simulink model "Feedforward_variations_Feb25_2017"  (R2016a)
settings: Solver=ode4  StartTime=0.0  StopTime=5  FixedStep=0.0001  RelTol=1e-3
values from neighbouring files (symbols this model uses):
  k = 10    [ff_demo_set_up.m]
  Kf = 1/(p+k)    (= 0.0666666666667)    [ff_demo_set_up.m]
  p = 5    [ff_demo_set_up.m]
libraries: simulink x4
settings Model: Creator=tac29  LastModifiedBy=DR_C

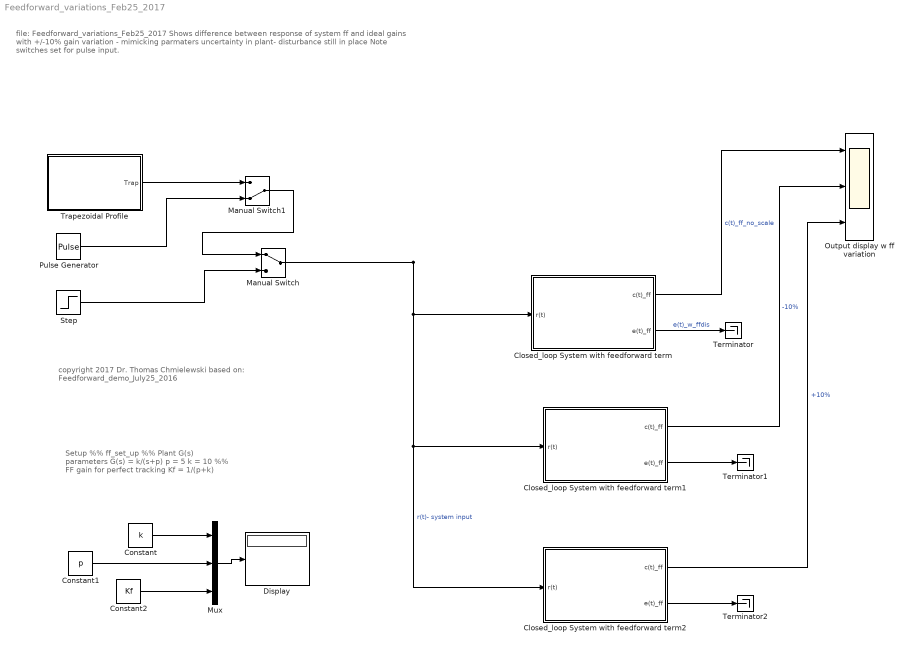
== system Feedforward_variations_Feb25_2017 ==
  note: file: Feedforward_variations_Feb25_2017
      | Shows difference between response of system ff and ideal gains with +/-10% gain variation - mimicking parmaters uncertainty in plant- disturbance still in place
      | Note switches set for pulse input.
  note: Setup
      | %% ff_set_up
      | %% Plant G(s) parameters   G(s) = k/(s+p)
      | p = 5
      | k = 10
      |
      | %% FF gain for perfect tracking
      | Kf = 1/(p+k)
  note: copyright 2017
      | Dr. Thomas Chmielewski
      | based on:
      | Feedforward_demo_July25_2016
  Closed_loop System with feedforward term : Subsystem
  Closed_loop System with feedforward term1 : Subsystem
  Closed_loop System with feedforward term2 : Subsystem
  Constant : Constant  Value=k
  Constant1 : Constant  Value=p
  Constant2 : Constant  Value=Kf
  Display : Display
  Manual Switch : ManualSwitch
  Manual Switch1 : ManualSwitch  CurrentSetting=0
  Mux : Mux  Inputs=3
  Output display w ff variation : Scope  NumInputPorts=3
  Pulse Generator : DiscretePulseGenerator  PulseType=Time based  Period=1  PulseWidth=50
  Step : Step  Time=0  SampleTime=0
  Terminator : Terminator
  Terminator1 : Terminator
  Terminator2 : Terminator
  Trapezoidal Profile : Subsystem
  wires:
  Step/1 -> Manual Switch/2
  Manual Switch/1 -> Closed_loop System with feedforward term2/1(r(t)), Closed_loop System with feedforward term1/1(r(t)), Closed_loop System with feedforward term/1(r(t))  "r(t)- system input"
  Mux/1 -> Display/1
  Constant2/1 -> Mux/3
  Constant1/1 -> Mux/2
  Constant/1 -> Mux/1
  Manual Switch1/1 -> Manual Switch/1
  Pulse Generator/1 -> Manual Switch1/2
  Trapezoidal Profile/1(Trap) -> Manual Switch1/1
  Closed_loop System with feedforward term/1(c(t)_ff) -> Output display w ff variation/1  "c(t)_ff_no_scale"
  Closed_loop System with feedforward term1/1(c(t)_ff) -> Output display w ff variation/2  "-10%"
  Closed_loop System with feedforward term2/1(c(t)_ff) -> Output display w ff variation/3  "+10%"
  Closed_loop System with feedforward term2/2(e(t)_ff) -> Terminator2/1
  Closed_loop System with feedforward term1/2(e(t)_ff) -> Terminator1/1
  Closed_loop System with feedforward term/2(e(t)_ff) -> Terminator/1  "e(t)_w_ffdis"

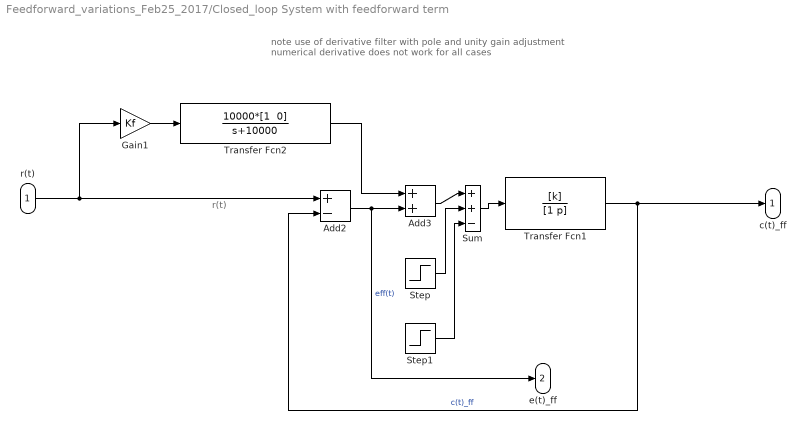
== system Feedforward_variations_Feb25_2017/Closed_loop System with feedforward term ==
  note: note use of derivative filter with pole and unity gain adjustment
      | numerical derivative does not work for all cases
  note: r(t)
  r(t) : Inport
  Add2 : Sum  Inputs=+-
  Add3 : Sum
  Gain1 : Gain  Gain=Kf
  Step : Step  Time=0  SampleTime=0
  Step1 : Step  Time=0  SampleTime=0
  Sum : Sum  Inputs=|++-
  Transfer Fcn1 : TransferFcn  Numerator=[k]  Denominator=[1 p]
  Transfer Fcn2 : TransferFcn  Numerator="10000*[1  0]"  Denominator=[1 10000]
  c(t)_ff : Outport
  e(t)_ff : Outport  Port=2
  wires:
  Add2/1 -> e(t)_ff/1, Add3/2  "eff(t)"
  Gain1/1 -> Transfer Fcn2/1
  Transfer Fcn1/1 -> c(t)_ff/1, Add2/2  "c(t)_ff"
  Transfer Fcn2/1 -> Add3/1
  r(t)/1 -> Add2/1, Gain1/1
  Add3/1 -> Sum/1
  Sum/1 -> Transfer Fcn1/1
  Step/1 -> Sum/2
  Step1/1 -> Sum/3

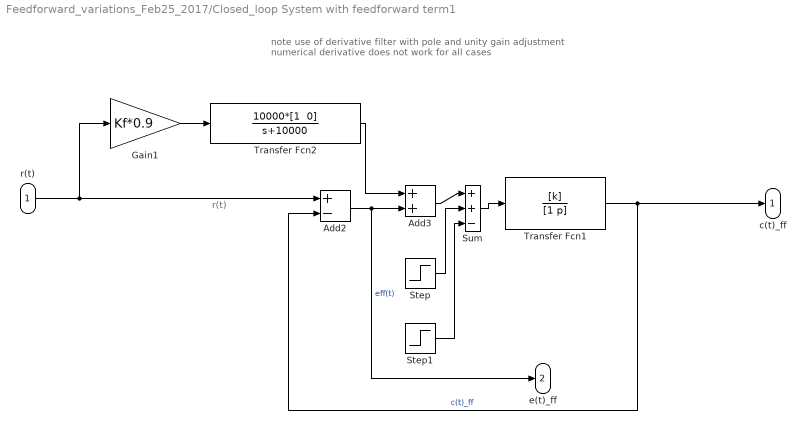
== system Feedforward_variations_Feb25_2017/Closed_loop System with feedforward term1 ==
  note: note use of derivative filter with pole and unity gain adjustment
      | numerical derivative does not work for all cases
  note: r(t)
  r(t) : Inport
  Add2 : Sum  Inputs=+-
  Add3 : Sum
  Gain1 : Gain  Gain=Kf*0.9
  Step : Step  Time=0  SampleTime=0
  Step1 : Step  Time=0  SampleTime=0
  Sum : Sum  Inputs=|++-
  Transfer Fcn1 : TransferFcn  Numerator=[k]  Denominator=[1 p]
  Transfer Fcn2 : TransferFcn  Numerator="10000*[1  0]"  Denominator=[1 10000]
  c(t)_ff : Outport
  e(t)_ff : Outport  Port=2
  wires:
  Add2/1 -> e(t)_ff/1, Add3/2  "eff(t)"
  Gain1/1 -> Transfer Fcn2/1
  Transfer Fcn1/1 -> c(t)_ff/1, Add2/2  "c(t)_ff"
  Transfer Fcn2/1 -> Add3/1
  r(t)/1 -> Add2/1, Gain1/1
  Add3/1 -> Sum/1
  Sum/1 -> Transfer Fcn1/1
  Step/1 -> Sum/2
  Step1/1 -> Sum/3

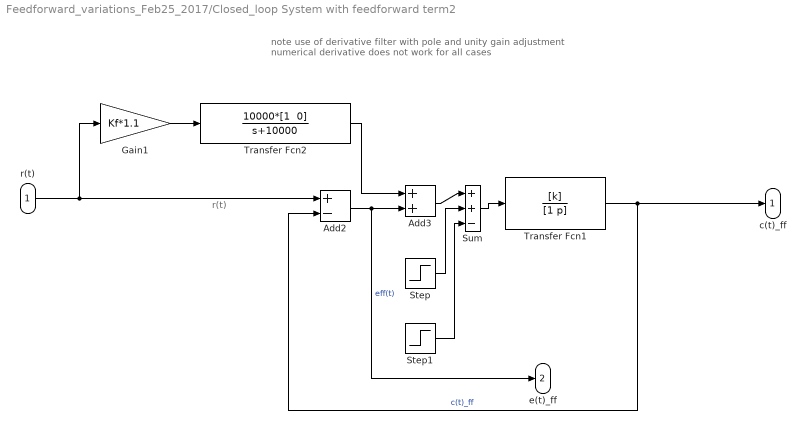
== system Feedforward_variations_Feb25_2017/Closed_loop System with feedforward term2 ==
  note: note use of derivative filter with pole and unity gain adjustment
      | numerical derivative does not work for all cases
  note: r(t)
  r(t) : Inport
  Add2 : Sum  Inputs=+-
  Add3 : Sum
  Gain1 : Gain  Gain=Kf*1.1
  Step : Step  Time=0  SampleTime=0
  Step1 : Step  Time=0  SampleTime=0
  Sum : Sum  Inputs=|++-
  Transfer Fcn1 : TransferFcn  Numerator=[k]  Denominator=[1 p]
  Transfer Fcn2 : TransferFcn  Numerator="10000*[1  0]"  Denominator=[1 10000]
  c(t)_ff : Outport
  e(t)_ff : Outport  Port=2
  wires:
  Add2/1 -> e(t)_ff/1, Add3/2  "eff(t)"
  Gain1/1 -> Transfer Fcn2/1
  Transfer Fcn1/1 -> c(t)_ff/1, Add2/2  "c(t)_ff"
  Transfer Fcn2/1 -> Add3/1
  r(t)/1 -> Add2/1, Gain1/1
  Add3/1 -> Sum/1
  Sum/1 -> Transfer Fcn1/1
  Step/1 -> Sum/2
  Step1/1 -> Sum/3

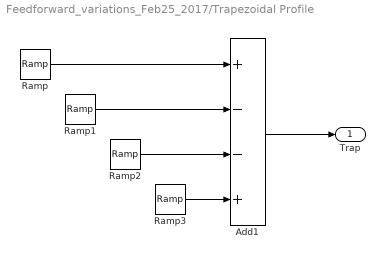
== system Feedforward_variations_Feb25_2017/Trapezoidal Profile ==
  Add1 : Sum  Inputs=+--+
  Ramp : simulink/Sources/Ramp  slope=1  start=0  X0=0
  Ramp1 : simulink/Sources/Ramp  slope=1  start=1  X0=0
  Ramp2 : simulink/Sources/Ramp  slope=1  start=2  X0=0
  Ramp3 : simulink/Sources/Ramp  slope=1  start=3  X0=0
  Trap : Outport
  wires:
  Ramp/1 -> Add1/1
  Ramp3/1 -> Add1/4
  Ramp2/1 -> Add1/3
  Ramp1/1 -> Add1/2
  Add1/1 -> Trap/1
